simulink model "sampleModel1399"  (R2023a)
settings: Solver=VariableStepAuto  StartTime=0.0  StopTime=10.0  RelTol=1e-3
libraries: hdlsllib x4, simulink x2
settings Model: Creator=user1  LastModifiedBy=user1

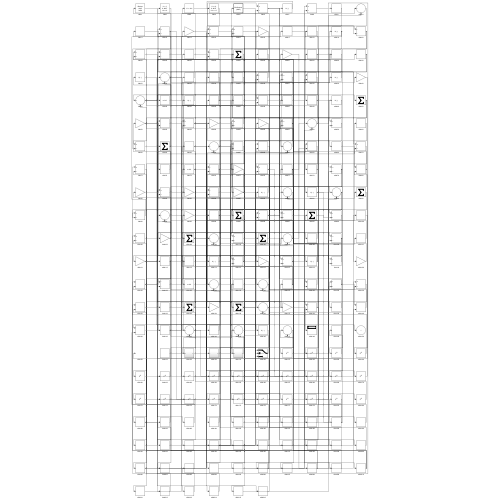
[thumbnail: Simulink's stored preview of the top-level diagram]
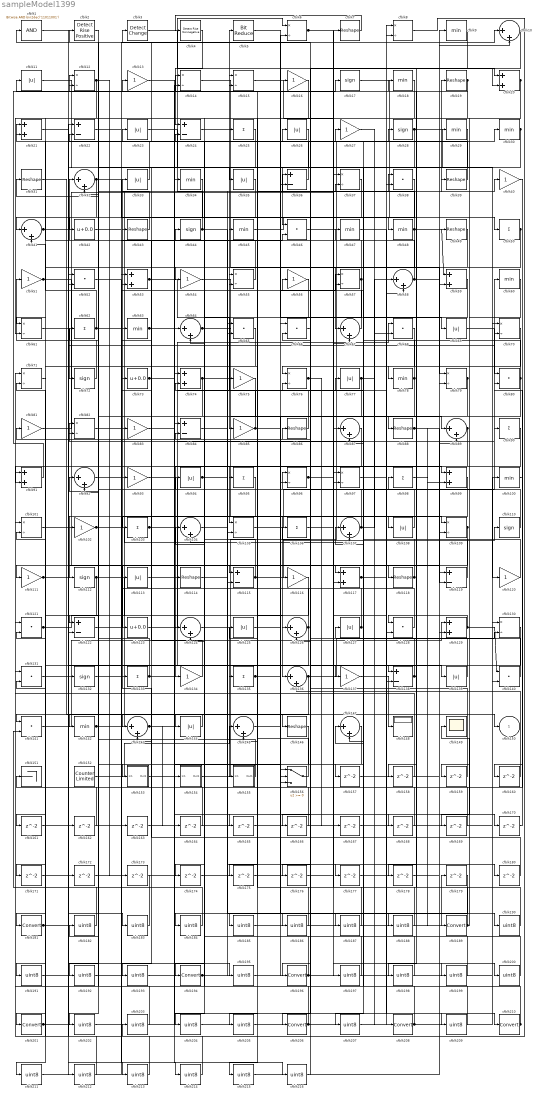
== system sampleModel1399 ==
  cfblk1 : simulink/Logic and Bit Operations/Bitwise Operator  logicop=AND  UseBitMask=on  BitMask=bin2dec('11011001')  BitMaskRealWorld=Stored Integer
      settings: LibrarySourceBlock=|
      | hdlsllib/Logic and Bit
      | Operations/Bitwise
      | Operator
  cfblk{10,32,41,58,64,67,87,89,92,104,107,124,126,136,143,145,147} (17 alike) : Sum  Inputs=|++
  cfblk{9,18,29..30,34,45,47..48,60,63,78,100,142} (13 alike) : MinMax
  cfblk{6,8,12,14..15,37,55,57,61,70..71,76,79,82,96..97,101,105,109,130} (20 alike) : Product  Inputs=*/  RndMeth=Zero  SaturateOnIntegerOverflow=on
  cfblk{13,16,27,40,51,54,56,75,81,83,85,93,102,111,116,120,134,137} (18 alike) : Gain
  cfblk{25,50,62,90,95,98,103,106,133,135} (10 alike) : Sum  Inputs=+
  cfblk{11,23,26,33,35,69,77,94,108,113,125,127,139,144} (14 alike) : Abs  SaturateOnIntegerOverflow=off
  cfblk{17,28,44,72,110,112,132} (7 alike) : Signum
  cfblk{7,19,31,39,43,49,86,88,114,118,146} (11 alike) : Reshape
  cfblk{22,24,36,84,115,119,122,138} (8 alike) : Sum  Inputs=+-
  cfblk{20..21,53,59,74,91,99,117,129} (9 alike) : Sum
  cfblk{38,46,52,65..66,68,80,121,128,131,140..141} (12 alike) : DotProduct  OutDataTypeStr=Inherit: Inherit via internal rule
  cfblk123 : Bias  Bias=0.0  SaturateOnIntegerOverflow=off
  cfblk148 : Display
  cfblk149 : Scope
  cfblk151 : Terminator
  cfblk152 : hdlsllib/Sources/Counter Limited  uplimit=7  tsamp=-1
  cfblk153 : Subsystem
      settings: LibrarySourceBlock=|
      | hdlsllib/Ports &
      | Subsystems/Subsystem
  cfblk154 : Subsystem
      settings: LibrarySourceBlock=|
      | hdlsllib/Ports &
      | Subsystems/Subsystem
  cfblk155 : Subsystem
      settings: LibrarySourceBlock=|
      | hdlsllib/Ports &
      | Subsystems/Subsystem
  cfblk156 : Switch  SaturateOnIntegerOverflow=off  InputSameDT=off
  cfblk{157..180} (24 alike) : Delay  SampleTime=1
  cfblk{181,189,194,196,201,206,208,210} (8 alike) : DataTypeConversion  SaturateOnIntegerOverflow=off  RndMeth=Floor
  cfblk{182..188,190..193,195,197..200,202..205,207,209,211..216} (28 alike) : DataTypeConversion  OutDataTypeStr=uint8  SaturateOnIntegerOverflow=off  RndMeth=Floor
  cfblk2 : hdlsllib/Logic and Bit Operations/Detect Rise Positive  vinit=0  OutDataTypeStr=boolean
  cfblk3 : simulink/Logic and Bit Operations/Detect Change  vinit=0  OutDataTypeStr=boolean
      settings: LibrarySourceBlock=|
      | hdlsllib/Logic and Bit
      | Operations/Detect
      | Change
  cfblk4 : hdlsllib/Logic and Bit Operations/Detect Rise Nonnegative  vinit=0  OutDataTypeStr=boolean
  cfblk42 : Bias  Bias=0.0  SaturateOnIntegerOverflow=off
  cfblk5 : hdlsllib/Logic and Bit Operations/Bit Reduce  mode=AND
  cfblk73 : Bias  Bias=0.0  SaturateOnIntegerOverflow=off
  cfblk150 : Outport  VectorParamsAs1DForOutWhenUnconnected=off
  wires:
  cfblk67/1 -> cfblk5/1
  cfblk123/1 -> cfblk26/1
  cfblk119/1 -> cfblk96/1
  cfblk58/1 -> cfblk32/1, cfblk10/2
  cfblk68/1 -> cfblk78/1
  cfblk17/1 -> cfblk105/1
  cfblk31/1 -> cfblk150/1
  cfblk142/1 -> cfblk44/1, cfblk45/1
  cfblk132/1 -> cfblk33/1
  cfblk95/1 -> cfblk112/1
  cfblk111/1 -> cfblk138/1, cfblk70/2, cfblk24/2
  cfblk51/1 -> cfblk123/1, cfblk195/1
  cfblk54/1 -> cfblk136/1
  cfblk34/1 -> cfblk201/1
  cfblk44/1 -> cfblk6/1, cfblk177/1
  cfblk139/1 -> cfblk81/1
  cfblk109/1 -> cfblk111/1, cfblk193/1
  cfblk154/1(Out1) -> cfblk28/1
  cfblk86/1 -> cfblk55/1
  cfblk10/1 -> cfblk88/1
  cfblk105/1 -> cfblk60/1
  cfblk74/1 -> cfblk109/1, cfblk122/1
  cfblk100/1 -> cfblk151/1
  cfblk113/1 -> cfblk90/1
  cfblk128/1 -> cfblk93/1
  cfblk115/1 -> cfblk110/1, cfblk21/2
  cfblk4/1 -> cfblk24/1
  cfblk92/1 -> cfblk108/1
  cfblk94/1 -> cfblk124/2, cfblk187/1
  cfblk141/1 -> cfblk129/1
  cfblk91/1 -> cfblk13/1
  cfblk18/1 -> cfblk115/1
  cfblk82/1 -> cfblk19/1
  cfblk63/1 -> cfblk126/1, cfblk156/2
  cfblk85/1 -> cfblk116/1, cfblk64/2
  cfblk127/1 -> cfblk43/1, cfblk15/1
  cfblk45/1 -> cfblk50/1
  cfblk64/1 -> cfblk89/1, cfblk170/1
  cfblk30/1 -> cfblk95/1, cfblk147/2
  cfblk155/1(Out1) -> cfblk92/1
  cfblk136/1 -> cfblk141/1, cfblk130/2
  cfblk89/1 -> cfblk105/2, cfblk91/2
  cfblk144/1 -> cfblk142/1
  cfblk53/1 -> cfblk85/1, cfblk117/2, cfblk96/2
  cfblk48/1 -> cfblk59/1, cfblk126/2, cfblk15/2
  cfblk102/1 -> cfblk107/2, cfblk62/1
  cfblk156/1 -> cfblk12/1
  cfblk75/1 -> cfblk143/1
  cfblk81/1 -> cfblk7/1
  cfblk14/1 -> cfblk79/1
  cfblk36/1 -> cfblk3/1
  cfblk76/1 -> cfblk166/1, cfblk167/1
  cfblk46/1 -> cfblk39/1
  cfblk24/1 -> cfblk67/1
  cfblk143/1 -> cfblk164/1, cfblk165/1
  cfblk57/1 -> cfblk54/1, cfblk104/2, cfblk75/1, cfblk21/1
  cfblk90/1 -> cfblk134/1
  cfblk134/1 -> cfblk63/1
  cfblk3/1 -> cfblk20/1
  cfblk33/1 -> cfblk2/1
  cfblk2/1 -> cfblk102/1
  cfblk135/1 -> cfblk180/1, cfblk190/1
  cfblk7/1 -> cfblk4/1
  cfblk117/1 -> cfblk58/2, cfblk157/1
  cfblk114/1 -> cfblk38/1
  cfblk112/1 -> cfblk154/1(In1), cfblk171/1
  cfblk20/1 -> cfblk158/1, cfblk159/1
  cfblk72/1 -> cfblk51/1
  cfblk69/1 -> cfblk80/1
  cfblk78/1 -> cfblk23/1, cfblk175/1
  cfblk131/1 -> cfblk132/1
  cfblk11/1 -> cfblk46/1
  cfblk1/1 -> cfblk118/1
  cfblk108/1 -> cfblk31/1
  cfblk120/1 -> cfblk82/1
  cfblk99/1 -> cfblk143/2
  cfblk27/1 -> cfblk208/1
  cfblk35/1 -> cfblk42/1
  cfblk41/1 -> cfblk30/1, cfblk137/1, cfblk29/1
  cfblk12/1 -> cfblk41/1, cfblk173/1
  cfblk5/1 -> cfblk69/1
  cfblk15/1 -> cfblk97/1
  cfblk83/1 -> cfblk210/1
  cfblk133/1 -> cfblk82/2, cfblk135/1
  cfblk124/1 -> cfblk155/1(In1)
  cfblk93/1 -> cfblk139/1
  cfblk25/1 -> cfblk113/1
  cfblk38/1 -> cfblk144/1
  cfblk6/1 -> cfblk20/2, cfblk119/2
  cfblk77/1 -> cfblk76/2, cfblk58/1, cfblk156/3, cfblk207/1
  cfblk19/1 -> cfblk12/2, cfblk61/2
  cfblk118/1 -> cfblk57/1, cfblk77/1, cfblk53/2
  cfblk71/1 -> cfblk181/1
  cfblk79/1 -> cfblk117/1, cfblk103/1
  cfblk39/1 -> cfblk25/1
  cfblk55/1 -> cfblk22/2
  cfblk138/1 -> cfblk86/1, cfblk178/1
  cfblk43/1 -> cfblk11/1
  cfblk22/1 -> cfblk14/1
  cfblk140/1 -> cfblk18/1
  cfblk84/1 -> cfblk99/1
  cfblk152/1 -> cfblk145/1
  cfblk80/1 -> cfblk47/1, cfblk198/1
  cfblk122/1 -> cfblk36/1
  cfblk49/1 -> cfblk52/2
  cfblk73/1 -> cfblk153/1(In1), cfblk46/2
  cfblk88/1 -> cfblk119/1, cfblk99/2
  cfblk125/1 -> cfblk68/1
  cfblk126/1 -> cfblk84/2, cfblk161/1, cfblk205/1
  cfblk103/1 -> cfblk38/2, cfblk216/1
  cfblk107/1 -> cfblk73/1, cfblk68/2
  cfblk23/1 -> cfblk120/1
  cfblk62/1 -> cfblk41/2, cfblk214/1
  cfblk153/1(Out1) -> cfblk114/1
  cfblk32/1 -> cfblk48/1, cfblk17/1, cfblk122/2
  cfblk96/1 -> cfblk40/1, cfblk128/2
  cfblk9/1 -> cfblk206/1
  cfblk66/1 -> cfblk196/1
  cfblk28/1 -> cfblk70/1, cfblk97/2
  cfblk137/1 -> cfblk148/1
  cfblk104/1 -> cfblk146/1
  cfblk110/1 -> cfblk74/2
  cfblk59/1 -> cfblk87/2
  cfblk98/1 -> cfblk189/1
  cfblk61/1 -> cfblk72/1
  cfblk21/1 -> cfblk35/1
  cfblk42/1 -> cfblk10/1
  cfblk16/1 -> cfblk194/1
  cfblk129/1 -> cfblk140/1, cfblk128/1
  cfblk121/1 -> cfblk124/1, cfblk183/1
  cfblk145/1 -> cfblk57/2
  cfblk50/1 -> cfblk61/1, cfblk188/1
  cfblk70/1 -> cfblk76/1
  cfblk157/1 -> cfblk129/2
  cfblk158/1 -> cfblk131/1
  cfblk159/1 -> cfblk1/1
  cfblk40/1 -> cfblk160/1
  cfblk160/1 -> cfblk136/2
  cfblk161/1 -> cfblk79/2
  cfblk162/1 -> cfblk22/1
  cfblk52/1 -> cfblk163/1
  cfblk163/1 -> cfblk87/1
  cfblk164/1 -> cfblk74/1
  cfblk165/1 -> cfblk138/2
  cfblk166/1 -> cfblk55/2
  cfblk167/1 -> cfblk140/2
  cfblk13/1 -> cfblk168/1
  cfblk168/1 -> cfblk32/2
  cfblk60/1 -> cfblk169/1
  cfblk169/1 -> cfblk107/1
  cfblk170/1 -> cfblk80/2
  cfblk171/1 -> cfblk14/2
  cfblk172/1 -> cfblk6/2
  cfblk173/1 -> cfblk141/2
  cfblk26/1 -> cfblk174/1
  cfblk174/1 -> cfblk115/2
  cfblk175/1 -> cfblk67/2
  cfblk130/1 -> cfblk176/1
  cfblk177/1 -> cfblk59/2
  cfblk178/1 -> cfblk109/2
  cfblk180/1 -> cfblk133/1
  cfblk181/1 -> cfblk162/1, cfblk213/1
  cfblk182/1 -> cfblk71/1
  cfblk183/1 -> cfblk71/2
  cfblk179/1 -> cfblk184/1
  cfblk184/1 -> cfblk53/1
  cfblk116/1 -> cfblk185/1
  cfblk185/1 -> cfblk179/1
  cfblk37/1 -> cfblk186/1
  cfblk186/1 -> cfblk125/1
  cfblk187/1 -> cfblk37/1
  cfblk188/1 -> cfblk37/2
  cfblk189/1 -> cfblk149/1, cfblk145/2
  cfblk190/1 -> cfblk98/1
  cfblk65/1 -> cfblk191/1
  cfblk191/1 -> cfblk172/1
  cfblk29/1 -> cfblk192/1
  cfblk192/1 -> cfblk65/1
  cfblk193/1 -> cfblk65/2
  cfblk194/1 -> cfblk156/1, cfblk36/2, cfblk89/2
  cfblk195/1 -> cfblk16/1
  cfblk196/1 -> cfblk130/1, cfblk94/1
  cfblk176/1 -> cfblk197/1
  cfblk197/1 -> cfblk66/1
  cfblk198/1 -> cfblk66/2
  cfblk106/1 -> cfblk199/1
  cfblk199/1 -> cfblk127/1
  cfblk47/1 -> cfblk200/1
  cfblk200/1 -> cfblk106/1
  cfblk201/1 -> cfblk84/1, cfblk64/1
  cfblk147/1 -> cfblk202/1
  cfblk202/1 -> cfblk34/1
  cfblk8/1 -> cfblk203/1
  cfblk203/1 -> cfblk121/1
  cfblk146/1 -> cfblk204/1
  cfblk204/1 -> cfblk8/1
  cfblk205/1 -> cfblk8/2
  cfblk206/1 -> cfblk121/2, cfblk104/1
  cfblk207/1 -> cfblk9/1
  cfblk208/1 -> cfblk147/1, cfblk91/1, cfblk100/1
  cfblk97/1 -> cfblk209/1
  cfblk209/1 -> cfblk27/1
  cfblk210/1 -> cfblk182/1, cfblk92/2, cfblk131/2
  cfblk87/1 -> cfblk211/1
  cfblk211/1 -> cfblk83/1
  cfblk101/1 -> cfblk212/1
  cfblk212/1 -> cfblk52/1
  cfblk213/1 -> cfblk101/1
  cfblk214/1 -> cfblk101/2
  cfblk56/1 -> cfblk215/1
  cfblk215/1 -> cfblk49/1
  cfblk216/1 -> cfblk56/1

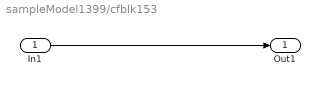
== system sampleModel1399/cfblk153 ==
  In1 : Inport
  Out1 : Outport
  wires:
  In1/1 -> Out1/1

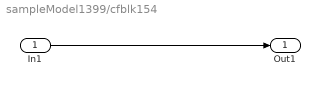
== system sampleModel1399/cfblk154 ==
  In1 : Inport
  Out1 : Outport
  wires:
  In1/1 -> Out1/1

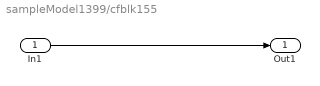
== system sampleModel1399/cfblk155 ==
  In1 : Inport
  Out1 : Outport
  wires:
  In1/1 -> Out1/1
